simulink model "Comax_Multiphysique"  (R2021a)
settings: Solver=VariableStepAuto  StartTime=0.0  StopTime=0.2  RelTol=1e-3
values from neighbouring files (symbols this model uses):
  g = 9.81    [param.m]
  Ke = 317    [param.m]
  kt = 0.108/(2*pi)    (= 0.0171887338539)    [param.m]
  Ma = 1.6+4*c    (= 3.64)    [param.m]
  Mm = 0    [param.m]
  R = 0.299    [param.m]
  Usat = 19.4    [param.m]
libraries: fl_lib x15, nesl_utility x4, ee_lib x1
settings Model: Creator=xpess  LastModifiedBy=xpess

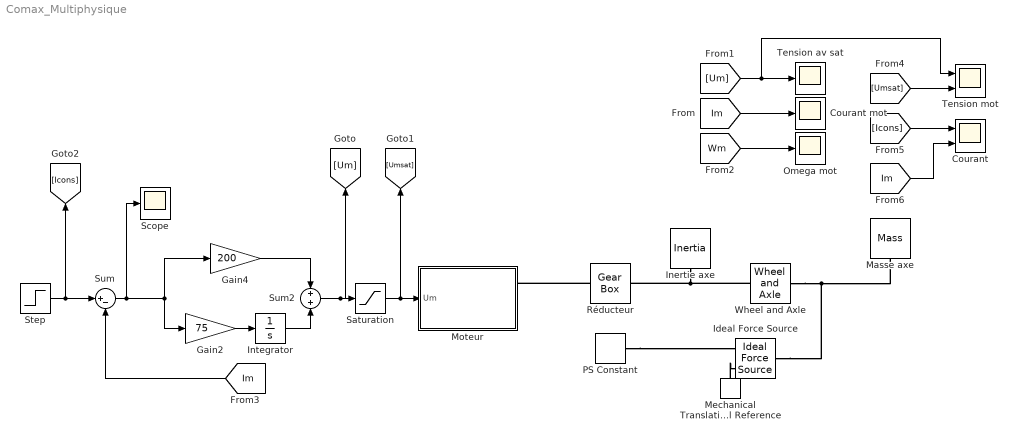
== system Comax_Multiphysique ==
  Courant : Scope  NumInputPorts=2
  Courant mot : Scope
  Gain2 : Gain  Gain=75
  Gain4 : Gain  Gain=200
  Ideal Force Source : fl_lib/Mechanical/Mechanical Sources/Ideal Force Source
  Inertie axe : fl_lib/Mechanical/Rotational Elements/Inertia  inertia=Ja g*cm^2  num_ports=foundation.enum.numPorts2.one  w_specify=off  w_priority=High  w=0 rad/s  w_nominal_specify=off  w_nominal_unit=rad/s  w_nominal_value=1  t_specify=off  t_priority=None  t=0 N*m  t_nominal_specify=off  t_nominal_unit=N*m  t_nominal_value=1
  Integrator : Integrator
  Masse axe : fl_lib/Mechanical/Translational Elements/Mass  mass=Ma kg  num_ports=foundation.enum.numPorts2.one  v_specify=off  v_priority=High  v=0 m/s  v_nominal_specify=off  v_nominal_unit=m/s  v_nominal_value=1  f_specify=off  f_priority=None  f=0 N  f_nominal_specify=off  f_nominal_unit=N  f_nominal_value=1
  Mechanical Translational Reference : fl_lib/Mechanical/Translational Elements/Mechanical Translational Reference
  Moteur : Subsystem
  Omega mot : Scope
  PS Constant : fl_lib/Physical Signals/Sources/PS Constant  constant=-g*(Ma+Mm)
  Réducteur : fl_lib/Mechanical/Mechanisms/Gear Box  ratio=k  t_in_specify=off  t_in_priority=None  t_in=0 N*m  t_in_nominal_specify=off  t_in_nominal_unit=N*m  t_in_nominal_value=1  t_out_specify=off  t_out_priority=None  t_out=0 N*m  t_out_nominal_specify=off  t_out_nominal_unit=N*m  t_out_nominal_value=1
  Saturation : Saturate  UpperLimit=Usat  LowerLimit=-Usat
  Scope : Scope
  Step : Step  Time=0  After=4.5  SampleTime=0
  Sum : Sum  Inputs=|+-
  Sum2 : Sum  Inputs=+|+
  Tension av sat : Scope
  Tension mot : Scope  NumInputPorts=2
  Wheel and Axle : fl_lib/Mechanical/Mechanisms/Wheel and Axle  R=kt m  or=1  t_specify=off  t_priority=None  t=0 N*m  t_nominal_specify=off  t_nominal_unit=N*m  t_nominal_value=1  f_specify=off  f_priority=None  f=0 N  f_nominal_specify=off  f_nominal_unit=N  f_nominal_value=1
  wires:
  [Wm] -> Omega mot/1
  [Im] -> Courant mot/1
  [Um] -> Tension mot/1, Tension av sat/1
  Gain2/1 -> Integrator/1
  Gain4/1 -> Sum2/1
  Sum2/1 -> [Um], Saturation/1
  Integrator/1 -> Sum2/2
  Step/1 -> [Icons], Sum/1
  Sum/1 -> Scope/1, Gain2/1, Gain4/1
  [Im] -> Sum/2
  Saturation/1 -> [Umsat], Moteur/1(Um)
  [Icons] -> Courant/1
  [Im] -> Courant/2
  [Umsat] -> Tension mot/2
  connections:
  Wheel and Axle/LConn1 -- Inertie axe/LConn1 -- Réducteur/RConn1
  Wheel and Axle/RConn1 -- Ideal Force Source/LConn1 -- Masse axe/LConn1
  Réducteur/LConn1 -- Moteur/RConn1
  Mechanical Translational Reference/LConn1 -- Ideal Force Source/RConn2
  PS Constant/RConn1 -- Ideal Force Source/RConn1

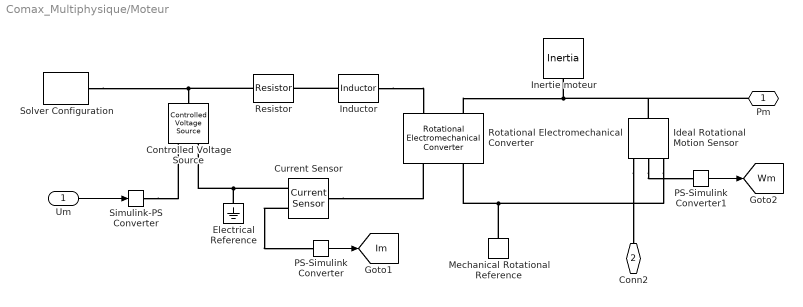
== system Comax_Multiphysique/Moteur ==
  Um : Inport
  Controlled Voltage Source : fl_lib/Electrical/Electrical Sources/Controlled Voltage Source
  Current Sensor : fl_lib/Electrical/Electrical Sensors/Current Sensor
  Electrical Reference : fl_lib/Electrical/Electrical Elements/Electrical Reference
  Ideal Rotational Motion Sensor : fl_lib/Mechanical/Mechanical Sensors/Ideal Rotational Motion Sensor  wrap_angle=simscape.enum.onoff.off  offset=0 rad
  Inductor : ee_lib/Passive/Inductor  l=L H  L_tol=20  enable_L_tol=0  tol_distribution=1  nSigma=4  r=0 Ohm  g=1e-9 1/Ohm  enable_operating_limits=0  operating_limit_action=2  max_working_current=1 A  power_rating=1 W  enable_faults=0  fault_action=1  lambdaPercent=50  k_faulted=0.9999  turnsShort=0  openCct=0  groundShort=0  groundShortG=0 1/Ohm  tau_fault=1e-3 s  enable_temporal_fault=0  t_fault=1 s  enable_behavioral_fault=0  max_permissible_voltage=100 V  n_fail_on_voltage=1  max_permissible_current=1 A  t_fail_on_current=1 s  i_L_specify=off  i_L_priority=High  i_L=0 A  i_L_nominal_specify=off  i_L_nominal_unit=A  i_L_nominal_value=1
  Inertie moteur : fl_lib/Mechanical/Rotational Elements/Inertia  inertia=Jm g*cm^2  num_ports=foundation.enum.numPorts2.one  w_specify=off  w_priority=High  w=0 rad/s  w_nominal_specify=off  w_nominal_unit=rad/s  w_nominal_value=1  t_specify=off  t_priority=None  t=0 N*m  t_nominal_specify=off  t_nominal_unit=N*m  t_nominal_value=1
  Mechanical Rotational Reference : fl_lib/Mechanical/Rotational Elements/Mechanical Rotational Reference
  PS-Simulink Converter : nesl_utility/PS-Simulink Converter  PhysicalDomain=network_engine_domain  SubClassName=ps_output  LeftPortType=input  RightPortType=output  PseudoPeriodic=off  Frequencies=[]  Unit=inherit  AffineConversion=off
      settings: SourceProductBaseCode=PW,SS
  PS-Simulink Converter1 : nesl_utility/PS-Simulink Converter  PhysicalDomain=network_engine_domain  SubClassName=ps_output  LeftPortType=input  RightPortType=output  PseudoPeriodic=off  Frequencies=[]  Unit=inherit  AffineConversion=off
      settings: SourceProductBaseCode=PW,SS
  Resistor : fl_lib/Electrical/Electrical Elements/Resistor  R=R Ohm  i_specify=off  i_priority=None  i=0 A  i_nominal_specify=off  i_nominal_unit=A  i_nominal_value=1  v_specify=off  v_priority=None  v=0 V  v_nominal_specify=off  v_nominal_unit=V  v_nominal_value=1
  Rotational Electromechanical Converter : fl_lib/Electrical/Electrical Elements/Rotational Electromechanical Converter  K=1/Ke V/rpm  i_specify=off  i_priority=None  i=0 A  i_nominal_specify=off  i_nominal_unit=A  i_nominal_value=1  v_specify=off  v_priority=None  v=0 V  v_nominal_specify=off  v_nominal_unit=V  v_nominal_value=1  t_specify=off  t_priority=None  t=0 N*m  t_nominal_specify=off  t_nominal_unit=N*m  t_nominal_value=1  w_specify=off  w_priority=None  w=0 rad/s  w_nominal_specify=off  w_nominal_unit=rad/s  w_nominal_value=1
  Simulink-PS Converter : nesl_utility/Simulink-PS Converter  PhysicalDomain=network_engine_domain  SubClassName=ps_input  LeftPortType=input  RightPortType=output  PseudoPeriodic=off  Frequencies=[]  NoiseDistribution=none  NoiseParameters=[]  Unit=1  AffineConversion=off  FilteringAndDerivatives=provide  SimscapeFilterOrder=1  InputFilterTimeConstant=0.001  UdotUserProvided=0
      settings: SourceProductBaseCode=PW,SS
  Solver Configuration : nesl_utility/Solver Configuration  PhysicalDomain=network_engine_domain  SubClassName=solver  LeftPortType=input  RightPortType=generic  Tones=[]  Harmonics=[]  SimulateNoise=off  Profile=off  UseLocalSampling=off  EnableSwitchedLinearOptims=on  FrequencyDomain=off  UseCCode=off  RelTol=0.001  AbsTol=1e-06  MinStep=1e-09  ToWorkspace=off  RevertToSquareIcSolve=off  NumHomotopyIterations=100  PhasorMode=off  PhasorModeNumHarmonics=1  DoDC=off  ResidualTolerance=1e-09  UseLocalSolver=off  LocalSolverChoice=NE_BACKWARD_EULER_ADVANCER  LocalSolverSampleTime=0.001  DoFixedCost=off  MaxNonlinIter=3  MaxModeIter=2  ComputeImpulses=off  ImpulseIterations=2  LinearAlgebra=auto  EquationFormulation=NE_TIME_EF  DelaysMemoryBudget=1024  AutomaticFiltering=on  FilteringTimeConstant=0.001  PartitionStorageMethod=AS_NEEDED  PartitionMemoryBudget=1024  PartitionMethod=ROBUST
      settings: SourceProductBaseCode=PW,SS
  Pm : PMIOPort  Side=Right
  Conn2 : PMIOPort  Port=2  Side=Right
  tag scope: Im=global, Wm=global
  wires:
  Um/1 -> Simulink-PS Converter/1
  PS-Simulink Converter/1 -> [Im]
  PS-Simulink Converter1/1 -> [Wm]
  connections:
  Mechanical Rotational Reference/LConn1 -- Ideal Rotational Motion Sensor/RConn1 -- Rotational Electromechanical Converter/RConn2
  Resistor/LConn1 -- Solver Configuration/RConn1 -- Controlled Voltage Source/LConn1
  Simulink-PS Converter/RConn1 -- Controlled Voltage Source/RConn1
  Inductor/LConn1 -- Resistor/RConn1
  Rotational Electromechanical Converter/LConn2 -- Pm/RConn1 -- Ideal Rotational Motion Sensor/LConn1 -- Inertie moteur/LConn1
  Electrical Reference/LConn1 -- Current Sensor/RConn2 -- Controlled Voltage Source/RConn2
  Inductor/RConn1 -- Rotational Electromechanical Converter/LConn1
  Current Sensor/LConn1 -- Rotational Electromechanical Converter/RConn1
  Ideal Rotational Motion Sensor/RConn3 -- Conn2/RConn1
  Ideal Rotational Motion Sensor/RConn2 -- PS-Simulink Converter1/LConn1
  Current Sensor/RConn1 -- PS-Simulink Converter/LConn1
